simulink model "Singlephase_INC_grid"  (R2023b)
settings: Solver=ode23t  StartTime=0.0  StopTime=4  FixedStep=1e-5  MaxStep=1e-4  RelTol=10e-4  EnableMultiTasking=on
undefined symbols (not defined in the file): Ion, Lithium, sigbuilder_block
libraries: spsFirstOrderFilterLib x13, spsSeriesRLCBranchLib x12, spsCurrentMeasurementLib x9, spsIGBTDiodeLib x7, spsVoltageMeasurementLib x5, spsPWMGeneratorDCDCLib x3, powerlib_extras x3, spsThreePhaseVIMeasurementLib x2, spsDiodeLib x2, spsGroundLib x2, spspowerguiLib x2, spsBatteryLib x1
settings Model: Creator=Administrator  LastModifiedBy=Chani
settings SolverCC: ZeroCrossControl=DisableAll  AlgebraicLoopSolver=TrustRegion
settings DataIOCC: LimitDataPoints=on  SaveFormat=Array  SignalLoggingSaveFormat=ModelDataLogs  ReturnWorkspaceOutputs=off
settings OptimizationCC: ExpressionDepthLimit=2147483647  LifeSpan=inf
settings DebuggingCC: UnderspecifiedInitializationDetection=Classic  MergeDetectMultiDrivingBlocksExec=none  SolverPrmCheckMsg=warning  FcnCallInpInsideContextMsg=warning  UnconnectedInputMsg=warning  UnconnectedOutputMsg=warning  UnconnectedLineMsg=warning  StateNameClashWarn=warning  SFUnexpectedBacktrackingDiag=warning  SFNoUnconditionalDefaultTransitionDiag=warning  SFExecutionAtInitializationDiag=none  ArithmeticOperatorsInVariantConditions=warning
settings HardwareCC: ProdBitPerPointer=32  ProdBitPerSizeT=32  ProdBitPerPtrDiffT=32  ProdLargestAtomicFloat=None  ProdIntDivRoundTo=Undefined  ProdEndianess=Unspecified  ProdWordSize=32  ProdHWDeviceType=32-bit Generic
settings ModelReferenceCC: EnableRefExpFcnMdlSchedulingChecks=on  PropagateSignalLabelsOutOfModel=off
settings SFSimCC: SimUseLocalCustomCode=off  CustomCodeUndefinedFunction=UseInterfaceOnly
settings RTWCC: RTWUseLocalCustomCode=off
settings CodeAppCC: StateflowObjectComments=on
settings GRTTargetCC: TargetLangStandard=C89/C90 (ANSI)  CombineOutputUpdateFcns=off  GRTInterface=on
settings ConfigComp: CovMetricSettings=dw  CovSaveCumulativeToWorkspaceVar=on  CovSaveSingleToWorkspaceVar=on  CovExternalEMLEnable=off
settings SimscapeCC: SimscapeNormalizeSystem=off

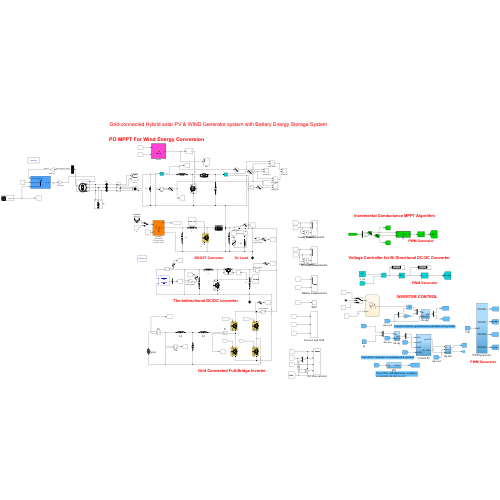
[thumbnail: Simulink's stored preview of the top-level diagram]
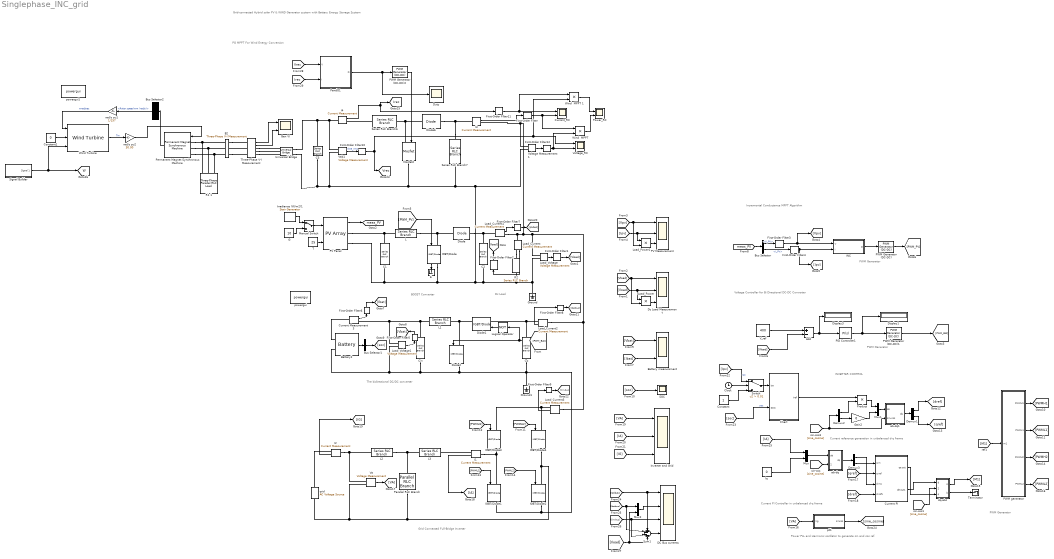
== system Singlephase_INC_grid ==
  note: Grid-connected Hybrid solar PV & WIND Generator system with Battery Energy Storage System
  note: Dc Load
  note: BOOST Converter
  note: Incremental Conductance MPPT Algorithm
  note: PWM Generator
  note: The bidirectional DC/DC converter
  note: PWM Generator
  note: Voltage Controller for Bi Directional DC-DC Converter
  note: Grid Connected Full-Bridge Inverter
  note: Current PI Controller in unbalanced d-q frame
  note: Power PLL and Harmonic oscillator to generate sin and cos ref.
  note: INVERTER CONTROL
  note: Current reference generation in unbalanced d-q frame
  note: PWM Generator
  note: PO MPPT For Wind Energy Conversion
  Add : Sum  Inputs=+-
  "B2 " : spsThreePhaseVIMeasurementLib/Three-Phase V-I Measurement  VoltageMeasurement=no  SetLabelV=on  LabelV=Vabc_B2  Vpu=off  VpuLL=off  CurrentMeasurement=no  SetLabelI=on  LabelI=Iabc_B2  Ipu=off  Pbase=100e6  Vbase=500e3  OutputType=Magnitude  PhasorSimulation=off  PSBequivalent=0
  Battery measurement : Scope  NumInputPorts=2
  Battery2 : spsBatteryLib/Battery  BatType=Lithium-Ion  ShowTempParam=off  ThermalPreset=no  ShowAgeParam=off  NomV=12*20  NomQ=48  SOC=50  Batt_Tr=0.0001  PresetModel=on  MaxQ=48  MinV=180  FullV=279.3569  Dis_rate=20.8696  R=0.05  Normal_OP=43.4087  expZone="[259.2926      2.358261]"  current=[1.5 3]  Units=Ampere-hour  Tci=20  NomT=20  T2=-30  MaxQ2=4.8  FullV2=7.1  Normal_OP2=5.72  expZone2="[6.58  1]"  Rca=0.6  ti=1000  Dp=0  Neq0=0  Tsim=1e6  Ta1=25  Qeol=5.4*0.9  Reol=0.013333*1.2  Char_age=[2.3478, 3]  Dis_age=[2.3478, 10]  N1=1500  N2=10500  N3=1000  N4=1400  Ta2=45  N5=950
      settings: LibrarySourceBlock=electricdrivelib/Extra Sources/Battery
  Bus Selector : BusSelector  OutputSignals=V_PV,I_PV
  Bus Selector1 : BusSelector  OutputSignals=SOC (%)  OutputAsBus=on
  Bus Selector2 : BusSelector  OutputSignals=Rotor speed wm (rad/s)
  C1 : spsSeriesRLCBranchLib/Series RLC Branch  LConnTagsString=__new0  RConnTagsString=__new0  BranchType=C  Resistance=1  Inductance=1e-3  SetiL0=off  InitialCurrent=0  Capacitance=4.8250e-05  Setx0=off  InitialVoltage=0  Measurements=None
  C2 : spsSeriesRLCBranchLib/Series RLC Branch  LConnTagsString=__new0  RConnTagsString=__new0  BranchType=C  Resistance=1  Inductance=1e-3  SetiL0=off  InitialCurrent=0  Capacitance=4.8250e-05  Setx0=off  InitialVoltage=0  Measurements=None
  C3 : spsSeriesRLCBranchLib/Series RLC Branch  LConnTagsString=__new0  RConnTagsString=__new0  BranchType=C  Resistance=0.001  Inductance=1e-3  SetiL0=off  InitialCurrent=0  Capacitance=4.8250e-05  Setx0=off  InitialVoltage=0  Measurements=None
  Chart : Stateflow chart  TreatAsAtomicUnit=on
  Cin : spsSeriesRLCBranchLib/Series RLC Branch  LConnTagsString=__new0  RConnTagsString=__new0  BranchType=C  Resistance=1  Inductance=3e-3  SetiL0=off  InitialCurrent=0  Capacitance=4.8250e-05  Setx0=off  InitialVoltage=0  Measurements=None
  Clock : Clock
  Co : spsSeriesRLCBranchLib/Series RLC Branch  LConnTagsString=__new0  RConnTagsString=__new0  BranchType=C  Resistance=1  Inductance=3e-3  SetiL0=off  InitialCurrent=0  Capacitance=4.8250e-05  Setx0=off  InitialVoltage=0  Measurements=None
  Constant : Constant
  Constant1 : Constant  Value=0
  Current Measurement3 : spsCurrentMeasurementLib/Current Measurement  PhasorSimulation=off  OutputType=Complex  PSBequivalent=0
  Current PI : Subsystem
  Current_RC : Scope  NumInputPorts=2
  DC Bus currents : Scope  NumInputPorts=4
  Dc Load Measurement : Scope  NumInputPorts=3
  Demux1 : Demux  Outputs=2
  Demux2 : Demux  Outputs=2
  Demux3 : Demux  Outputs=2
  Diode : spsDiodeLib/Diode  Ron=0.001  Lon=0  Vf=0.8  IC=0  UseSnubber=off  Rs=500  Cs=250e-9  Measurements=off
  Diode1 : spsIGBTDiodeLib/IGBT//Diode  Ron=1e-3  Rs=1e5  Cs=inf  Measurements=on
  Diode2 : spsIGBTDiodeLib/IGBT//Diode  Ron=1e-3  Rs=1e5  Cs=inf  Measurements=on
  Diode6 : spsDiodeLib/Diode  Ron=0.001  Lon=0  Vf=0.8  IC=0  UseSnubber=0  Rs=500  Cs=250e-9  Measurements=off
  Display1 : Display
  Display3 : Display
  Duty : Scope
  E : Terminator
  First-Order Filter{,1..12} (13 alike) : spsFirstOrderFilterLib/First-Order Filter  FilterType=Lowpass  Tc=10e-3  Ts=0  Initialize=on  Vac_Init=[0, 0, 60]  Vdc_Init=0  PlotResponse=off  FreqRange="[0,  200,  1]"
  G : Constant  Value=10
  Gain2 : Gain  Gain=0
  Gen VI : Scope  NumInputPorts=2
  Ground : spsGroundLib/Ground  LConnTagsString=a
  Ground1 : spsGroundLib/Ground  LConnTagsString=a
  I{1..4} (4 alike) : spsCurrentMeasurementLib/Current Measurement  PhasorSimulation=off  OutputType=Complex  PSBequivalent=0
  IGBT/Diode{,1..4} (5 alike) : spsIGBTDiodeLib/IGBT//Diode  Ron=1e-3  Rs=1e5  Cs=inf  Measurements=on
  INC : MATLAB Function  TreatAsAtomicUnit=on
  Inverter and Grid : Scope  NumInputPorts=3
  Iq : Constant  Value=0
  Irradiance (W/m2)1 : spsStairGeneratorLib/Stair Generator  t=[0, 0.3, 0.6,0.9, 1.2]  e=[1,0.5, 0.01, 0.5, 1]*1000  Ts=0.0001
  L : spsSeriesRLCBranchLib/Series RLC Branch  LConnTagsString=__new0  RConnTagsString=__new0  BranchType=L  Resistance=1  Inductance=0.1164  SetiL0=off  InitialCurrent=0  Capacitance=1e-6  Setx0=off  InitialVoltage=0  Measurements=None
  L1 : spsSeriesRLCBranchLib/Series RLC Branch  LConnTagsString=__new0  RConnTagsString=__new0  BranchType=L  Resistance=.25  Inductance=0.1164  SetiL0=off  InitialCurrent=0  Capacitance=1e-6  Setx0=off  InitialVoltage=0  Measurements=None
  L2 : spsSeriesRLCBranchLib/Series RLC Branch  LConnTagsString=__new0  RConnTagsString=__new0  BranchType=L  Resistance=0.001  Inductance=0.72e-3  SetiL0=off  InitialCurrent=0  Capacitance=1e-6  Setx0=off  InitialVoltage=0  Measurements=None
  L3 : spsSeriesRLCBranchLib/Series RLC Branch  LConnTagsString=__new0  RConnTagsString=__new0  BranchType=L  Resistance=1.5  Inductance=6.6e-3  SetiL0=off  InitialCurrent=0  Capacitance=1e-6  Setx0=off  InitialVoltage=0  Measurements=None
  Load_Current{,1..3} (4 alike) : spsCurrentMeasurementLib/Current Measurement  PhasorSimulation=off  OutputType=Complex  PSBequivalent=0
  Load_Power : Product  RndMeth=Zero
  Load_Power1 : Product  RndMeth=Zero
  Load_Voltage : spsVoltageMeasurementLib/Voltage Measurement  PhasorSimulation=off  OutputType=Complex  PSBequivalent=0
  Load_Voltage1 : spsVoltageMeasurementLib/Voltage Measurement  PhasorSimulation=off  OutputType=Complex  PSBequivalent=0
  Logical Operator : Logic  Operator=NOT  AllPortsSameDT=off  OutDataTypeStr=boolean
  Manual Switch : ManualSwitch
  Mosfet2 : spsMosfetLib/Mosfet  Ron=0.1  Lon=0  Rd=0.01  Vfd=0.8  IC=0  Rs=1e5  Cs=inf  Measurements=off
  Mux : Mux  Inputs=2
  Mux1 : Mux  Inputs=2
  Mux2 : Mux  Inputs=2
  PID Controller1 : slpidlib/PID Controller  Controller=PI  Form=Parallel  TimeDomain=Continuous-time  UseExternalTs=off  SampleTime=-1  IntegratorMethod=Forward Euler  FilterMethod=Forward Euler  ControllerParametersSource=internal  P=0.00001  I=0.05  UseKiTs=off  D=0  N=100  UseFilter=on  TunerSelectOption=Transfer Function Based (PID Tuner App)  InitialConditionSource=internal  InitialConditionForIntegrator=0  InitialConditionForFilter=0  DifferentiatorICPrevScaledInput=0  ExternalReset=none  TrackingMode=off  Kt=1  LimitOutput=off  SatLimitsSource=internal  UpperSaturationLimit=inf  LowerSaturationLimit=-inf  LinearizeAsGain=on  AntiWindupMode=none  Kb=1  LimitIntegrator=off  UpperIntegratorSaturationLimit=inf  LowerIntegratorSaturationLimit=-inf  POutMin=[]  POutMax=[]  IOutMin=[]  IOutMax=[]  DOutMin=[]  DOutMax=[]  NOutMin=[]  NOutMax=[]  SumOutMin=[]  SumOutMax=[]  SaturationOutMin=[]  SaturationOutMax=[]  PParamMin=[]  PParamMax=[]  IParamMin=[]  IParamMax=[]  DParamMin=[]  DParamMax=[]  NParamMin=[]  NParamMax=[]  KbParamMin=[]  KbParamMax=[]  KtParamMin=[]  KtParamMax=[]  KbOutMin=[]  KbOutMax=[]  KtOutMin=[]  KtOutMax=[]  IntegratorOutMin=[]  IntegratorOutMax=[]  FilterOutMin=[]  FilterOutMax=[]  SumI1OutMin=[]  SumI1OutMax=[]  SumI2OutMin=[]  SumI2OutMax=[]  SumI3OutMin=[]  SumI3OutMax=[]  SumI4OutMin=[]  SumI4OutMax=[]  SumDOutMin=[]  SumDOutMax=[]  DifferentiatorOutMin=[]  DifferentiatorOutMax=[]  FilterDiffOutCoefMin=[]  FilterDiffOutCoefMax=[]  ReciprocalOutMin=[]  ReciprocalOutMax=[]  SumDenOutMin=[]  SumDenOutMax=[]  SumNumOutMin=[]  SumNumOutMax=[]  DivideOutMin=[]  DivideOutMax=[]  UdiffTsProdOutMin=[]  UdiffTsProdOutMax=[]  NTsProdOutMin=[]  NTsProdOutMax=[]  UintegralTsProdOutMin=[]  UintegralTsProdOutMax=[]  UngainTsProdOutMin=[]  UngainTsProdOutMax=[]  ClampingZeroOutDataTypeStr=Inherit: Inherit via back propagation  ClampingZeroOutMin=[]  ClampingZeroOutMax=[]  FilterDenConstantOutDataTypeStr=Inherit: Inherit via back propagation  FilterDenConstantOutMin=[]  FilterDenConstantOutMax=[]  PCopyOutDataTypeStr=Inherit: Inherit via back propagation  PCopyOutMin=[]  PCopyOutMax=[]  NCopyOutDataTypeStr=Inherit: Inherit via back propagation  NCopyOutMin=[]  NCopyOutMax=[]  IntegratorContinuousStateAttributes=''  IntegratorStateMustResolveToSignalObject=off  IntegratorRTWStateStorageClass=Auto  FilterContinuousStateAttributes=''  FilterStateMustResolveToSignalObject=off  FilterRTWStateStorageClass=Auto  ParallelPVariant=InternalParameters  IdealPVariant=Disabled  IVariant=InternalParameters  DVariant=Disabled  IntegratorVariant=Continuous  SatVariant=Disabled  AWVariant=Passthrough  PCopyVariant=Disabled  TRVariant=Disabled  FdbkBlocksVariant=Forward  IdealPFdbkVariant=Disabled  SatFdbkVariant=Disabled  DerivativeFilterVariant=Disabled  NVariant=Disabled  NCopyVariant=Disabled_SignalSpec  FilterICVariant=Disabled  IntegratorICVariant=InternalICs  ExternalResetVariant=Disabled  TRSumVariant=Passthrough  SumFdbkVariant=Disabled  SumVariant=Sum_PI  TsampFilterVariant=InternalTs  TsampNgainVariant=Passthrough  TsampIntegralVariant=Disabled_SignalSpec  ExternalSaturationOutDataTypeStr=Inherit: Same as second input
  PV Measurement : Scope  NumInputPorts=3
  PV Panel : spsPVArrayLib/PV Array  Npar=1  Nser=8  PlotType=array @ 25 deg.C & specified irradiances  S_vec="[ 1000 800  600  400 ]"  Temp_C_vec="[ 45 25  ]"  ModuleName=User-defined  PlotWhenSelected=off  Pm=250.205  Ncell=60  Voc=37.3  Isc=8.66  Vm=30.7  Im=8.15  beta_Voc_pc=-0.36901  alpha_Isc_pc=0.086998  beta_Voc=-0.13764  alpha_Isc=0.007534  IL=8.7062  I0=4.1579e-10  nI=1.0189  Rsh=240.6015  Rs=0.23732  RobustModel=off  RobustCellTemperature=313.3991  BAL=on  Tc=1e-6  Tfilter=1e-5
      settings: AttributesFormatString=|
      | %<ModuleName>
      | %<Nser>-module string
      | %<Npar> parallel strings
  PWM Generator (DC-DC) : spsPWMGeneratorDCDCLib/PWM Generator (DC-DC)  Fsw=10000  Ts=0
  PWM Generator (DC-DC)1 : spsPWMGeneratorDCDCLib/PWM Generator (DC-DC)  Fsw=10000  Ts=0
  PWM Generator (DC-DC)2 : spsPWMGeneratorDCDCLib/PWM Generator (DC-DC)  Fsw=5000  Ts=0
  PWM generator : Subsystem
  PandO1 : MATLAB Function  TreatAsAtomicUnit=on
  Parallel RLC Branch : spsParallelRLCBranchLib/Parallel RLC Branch  LConnTagsString=a  RConnTagsString=__new0  BranchType=C  Resistance=1  Inductance=1e-3  SetiL0=off  InitialCurrent=0  Capacitance=6.91e-6  Setx0=off  InitialVoltage=0  Measurements=None
  Permanent Magnet Synchronous Machine : spsPermanentMagnetSynchronousMachineLib/Permanent Magnet Synchronous Machine  NbPhases=3  FluxDistribution=Sinusoidal  RotorType=Round  MechanicalLoad=Torque Tm  PresetModel="06:  10 Nm 300 Vdc 2300 RPM - 14.2 Nm"  ShowDetailedParameters=on  MeasurementBus=off  Resistance=0.4578  Inductance=8.5e-3  dqInductances=[8.5e-3,8.5e-3]  La=0.00334  MachineConstant=Flux linkage established by magnets (V.s)  Flux=0.171  VoltageCst=124.0639  TorqueCst=1.026  Flat=120  Mechanical=[0.001469 0.0003035 4 0]  PolePairs=4  InitialConditions=[0,0, 0,0]  InitialConditions5ph=[0 0 0 0 0 0]  RefAngle=90 degrees behind phase A axis (modified Park)  IterativeDiscreteModel=Trapezoidal non iterative  TsBlock=-1  TsPowergui=0
  Power_RC : Scope  NumInputPorts=2
  Product : Product  RndMeth=Zero
  R1 1 : spsThreePhaseParallelRLCLoadLib/Three-Phase Parallel RLC Load  LConnTagsString=A|B|C  Configuration=Y (grounded)  NominalVoltage=220  Vabc=[1e3 1e3 1e3]  Vabcp=[1e3 1e3 1e3]  NominalFrequency=50  UnbalancedPower=off  ActivePower=1000  InductivePower=0  CapacitivePower=0  Pabc=[9e3 9e3 9e3]  QLabc=[100 90 110]  QCabc=[100 90 110]  Pabcp=[10e3 9e3 11e3]  QLabcp=[100 90 110]  QCabcp=[100 90 110]  Measurements=None  LoadType=constant Z
  R2 : spsSeriesRLCBranchLib/Series RLC Branch  LConnTagsString=__new0  RConnTagsString=__new0  BranchType=R  Resistance=160  Inductance=1e-3  SetiL0=off  InitialCurrent=0  Capacitance=1e-6  Setx0=off  InitialVoltage=0  Measurements=None
  SOC : Scope
  Series RLC Branch6 : spsSeriesRLCBranchLib/Series RLC Branch  LConnTagsString=__new0  RConnTagsString=__new0  BranchType=L  Resistance=1  Inductance=0.1164  SetiL0=off  InitialCurrent=0  Capacitance=1e-6  Setx0=off  InitialVoltage=0  Measurements=None
  Series RLC Branch7 : spsSeriesRLCBranchLib/Series RLC Branch  LConnTagsString=__new0  RConnTagsString=__new0  BranchType=C  Resistance=110  Inductance=1e-3  SetiL0=off  InitialCurrent=0  Capacitance=4.8250e-05  Setx0=off  InitialVoltage=0  Measurements=None
  Signal Builder : Subsystem  Tag=STV Subsys  LoadFcn=sigbuilder_block('load');  StartFcn=sigbuilder_block('start');  StopFcn=sigbuilder_block('stop');  ClipboardFcn=sigbuilder_block('clipboard');  mask(Sigbuilder block){tuvar=[0:10]}
      mask help: Simulink:masks:SigbuilderBlock_MD
      mask init:
      | if ~strcmp(get_param(bdroot(gcbh),'SimulationStatus'),'stopped') tuvar = sigbuilder_block('maskInit'); end
      settings: CopyFcn=sigbuilder_block('copy');  DeleteFcn=sigbuilder_block('delete');  ModelCloseFcn=sigbuilder_block('modelClose');  PreSaveFcn=sigbuilder_block('preSave');  PauseFcn=sigbuilder_block('pause');  ContinueFcn=sigbuilder_block('continue');  NameChangeFcn=sigbuilder_block('namechange');  OpenFcn=sigbuilder_block('open',[333.75 182.25 550.5 359.25 ]);  CloseFcn=sigbuilder_block('close');
      mask Display: plot(0, 0, 100, 100,[2, 2, 32, 32, 2], [68, 8, 8, 68, 68],[32, 2], [38, 38], [32, 19, 2],[53, 60, 44], [32, 17, 17, 2],[16, 16, 31, 31]);txt = getActiveGroup(gcbh);text(2, 100, txt,'verticalAlignment', 'top');
  Sum1 : Sum  Inputs=+---
  Switch : Switch  Criteria=u2 > Threshold  Threshold=0.01  SaturateOnIntegerOverflow=off  InputSameDT=off
  T : Constant  Value=25
  Terminator : Terminator
  Three-Phase V-I Measurement : spsThreePhaseVIMeasurementLib/Three-Phase V-I Measurement  VoltageMeasurement=phase-to-phase  SetLabelV=off  LabelV=Vabc  Vpu=off  VpuLL=off  CurrentMeasurement=yes  SetLabelI=off  LabelI=Iabc  Ipu=off  Pbase=100e6  Vbase=500e3  OutputType=Complex  PhasorSimulation=off  PSBequivalent=0
  Universal Bridge : spsUniversalBridgeLib/Universal Bridge  Arms=3  SnubberResistance=1e5  SnubberCapacitance=inf  Device=Diodes  Ron=1e-3  Lon=0  ForwardVoltages="[  0  0  ]"  ForwardVoltage=0.8  GTOparameters=[ 10e-6 , 20e-6 ]  IGBTparameters=[ 1e-6 , 2e-6 ]  Measurements=None  Measurements_2=None  converterType=Rectifier
  V_ref : Constant  Value=400
  Va : spsVoltageMeasurementLib/Voltage Measurement  PhasorSimulation=off  OutputType=Complex  PSBequivalent=0
  Vab1 : spsVoltageMeasurementLib/Voltage Measurement  PhasorSimulation=off  OutputType=Complex  PSBequivalent=0
  Voltage Measurement1 : spsVoltageMeasurementLib/Voltage Measurement  PhasorSimulation=off  OutputType=Complex  PSBequivalent=0
  Voltage_RC : Scope  NumInputPorts=2
  "Wind  MPPT " : Product
  Wind  MPPT 1 : Product
  Wind Turbine : spsWindTurbineLib/Wind Turbine  Pnom=2.5e3  Pelec_base=2.5e3/0.9  wind_base=12  P_wind_base=1  speed_nom=1.3  pitch_angle=0  c1_c6="[0.51763          116          0.4            5           21     0.006795]"  cp_nom=0.48  lambda_nom=8.1
  ab-dq : Subsystem
  ab-dq1 : Subsystem
  dq-abc : Subsystem
  grid : spsACVoltageSourceLib/AC Voltage Source  Amplitude=230*sqrt(2)  Phase=0  Frequency=50  SampleTime=0  Measurements=None  BusType=swing  Pref=1e3  Qref=500  Qmin=-inf  Qmax=+inf
  pll1 : Subsystem
  powergui : spspowerguiLib/powergui  Priority=1  SimulationMode=Continuous  SampleTime=1e-6  frequency=60  Iterations=50  frequencyindice=0  Pbase=100e6  ErrMax=1e-4  UnitsV=kV  UnitsW=MW  buscounter=0  FunctionMessages=off  echomessages=off  EnableUseOfTLC=off  CurrentSourceSwitches=off  DisableSnubberDevices=off  DisableRonSwitches=off  DisableVfSwitches=off  DisplayEquations=off  AutomaticDiscreteSolvers=off  SolverType=Tustin/Backward Euler (TBE)  Interpol=off  ExternalGateDelay=off  methode=off  Ts=100  x0status=blocks  SPID=on  SwTol=0  HookPort=off  NonlinearTolerance=1e-4  nMaxIteration=100  ContinueOnMaxIteration=off  RestoreLinks=warning  ResistiveCurrentMeasurement=off  Frange=[0:2:500]  Ylog=off  Xlog=on  ShowGrid=off  save=off  variable=ZData  structure=0  ZoomFFT=off  StartTime=0.0  cycles=1  DisplayStyle=1  fundamental=60  FreqAxis=off  MaxFrequency=1000  frequencyindicesteady=1  RmsSteady=1  display=off
  powergui1 : spspowerguiLib/powergui  Priority=1  SimulationMode=Continuous  SampleTime=50e-6  frequency=60  Iterations=50  frequencyindice=0  Pbase=100e6  ErrMax=1e-4  UnitsV=kV  UnitsW=MW  buscounter=0  FunctionMessages=off  echomessages=off  EnableUseOfTLC=off  CurrentSourceSwitches=off  DisableSnubberDevices=off  DisableRonSwitches=off  DisableVfSwitches=off  DisplayEquations=off  AutomaticDiscreteSolvers=off  SolverType=Tustin/Backward Euler (TBE)  Interpol=off  ExternalGateDelay=off  methode=off  Ts=100  x0status=blocks  SPID=on  SwTol=0  HookPort=off  NonlinearTolerance=1e-4  nMaxIteration=100  ContinueOnMaxIteration=off  RestoreLinks=warning  ResistiveCurrentMeasurement=off  Frange=[0:2:500]  Ylog=off  Xlog=on  ShowGrid=off  save=off  variable=ZData  structure=0  ZoomFFT=off  StartTime=0.0  cycles=1  DisplayStyle=1  fundamental=60  FreqAxis=off  MaxFrequency=1000  frequencyindicesteady=1  RmsSteady=1  display=off
  rad/s pu1 : Gain  Gain=1/157  SaturateOnIntegerOverflow=on  OutDataTypeStr=Inherit: Same as input  ParamDataTypeStr=Inherit: Same as input
  rad/s pu2 : Gain  Gain=30.00  SaturateOnIntegerOverflow=on  OutDataTypeStr=Inherit: Same as input  ParamDataTypeStr=Inherit: Same as input
  tag scope: Irec=global, Vrec=global, W=global, meas_PV=global
  wires:
  T/1 -> PV Panel/2
  IGBT/Diode/1 -> E/1
  PV Panel/1 -> [meas_PV]
  [meas_PV] -> Bus Selector/1
  Bus Selector/2 -> First-Order Filter4/1  "<I_PV>"
  Bus Selector/1 -> First-Order Filter3/1  "<V_PV>"
  INC/1(D) -> PWM Generator (DC-DC)/1
  Manual Switch/1 -> PV Panel/1
  Irradiance (W/m2)1/1 -> Manual Switch/1
  G/1 -> Manual Switch/2
  V_ref/1 -> Add/1
  [Vload] -> Add/2
  Load_Voltage/1 -> First-Order Filter1/1
  Load_Current/1 -> First-Order Filter2/1
  First-Order Filter3/1 -> [Vpv], INC/1(V)
  First-Order Filter4/1 -> [Ipv], INC/2(I)
  Battery2/1 -> Bus Selector1/1
  Logical Operator/1 -> Diode1/1
  First-Order Filter2/1 -> [Iload]
  First-Order Filter1/1 -> [Vload]
  PWM Generator (DC-DC)/1 -> [PWM_PV]
  [PWM_PV] -> IGBT/Diode/1
  PWM Generator (DC-DC)1/1 -> [PWM_Bat]
  [PWM_Bat] -> Logical Operator/1, Diode2/1
  Current Measurement3/1 -> First-Order Filter6/1
  Load_Voltage1/1 -> First-Order Filter5/1
  Bus Selector1/1 -> [soc]
  [Vpv] -> Load_Power1/2, PV Measurement/1
  [Ipv] -> Load_Power1/1, PV Measurement/2
  Load_Power1/1 -> PV Measurement/3
  [Ibat] -> Battery measurement/2
  [Vbat] -> Battery measurement/1
  First-Order Filter6/1 -> [Ibat]
  First-Order Filter5/1 -> [Vbat]
  [Vload] -> Load_Power/2, Dc Load Measurement/1
  [Iload] -> Load_Power/1, Dc Load Measurement/2
  Load_Power/1 -> Dc Load Measurement/3
  [PWML1] -> IGBT/Diode1/1
  [PWML2] -> IGBT/Diode2/1
  [PWMH1] -> IGBT/Diode3/1
  [PWMH2] -> IGBT/Diode4/1
  Mux1/1 -> ab-dq1/1(ab)
  PWM generator/1(PWMH1) -> [PWMH1]
  ab-dq/1(dq) -> Demux3/1
  [VA] -> pll1/1(Vg)
  Current PI/1(qe out) -> dq-abc/3(q)
  Gain2/1 -> Mux1/2
  Product/1 -> Mux1/1
  Demux1/2 -> [qref]
  [dref] -> Current PI/4(d ref1)
  Demux2/2 -> Gain2/1
  Demux3/2 -> Current PI/1(q in)
  PWM generator/4(PWML2) -> [PWML2]
  [qref] -> Current PI/2(q ref)
  Demux2/1 -> Product/2
  [sine_cosine] -> ab-dq1/2(sin-cos), Demux2/1
  Iq/1 -> Mux/2
  Demux1/1 -> [dref]
  [sine_cosine] -> dq-abc/2(sin-cos)
  ab-dq1/1(dq) -> Demux1/1
  dq-abc/1(a) -> [M1]
  Mux/1 -> ab-dq/1(ab)
  [sine_cosine] -> ab-dq/2(sin-cos)
  PWM generator/3(PWMH2) -> [PWMH2]
  [IA] -> Mux/1
  Current PI/2(de out1) -> dq-abc/1(d)
  Demux3/1 -> Current PI/3(d in1)
  PWM generator/2(PWML1) -> [PWML1]
  pll1/1(sincos) -> [sine_cosine]
  [M1] -> PWM generator/1(m1)
  dq-abc/2(b) -> Terminator/1
  Va/1 -> [VA]
  I1/1 -> [IA]
  I2/1 -> [IG]
  [VA] -> Inverter and Grid/1
  [IA] -> Inverter and Grid/2
  [IG] -> Inverter and Grid/3
  [soc] -> SOC/1
  Add/1 -> PID Controller1/1, Display3/1
  PID Controller1/1 -> Display1/1, PWM Generator (DC-DC)1/1
  Load_Current1/1 -> First-Order Filter7/1
  Load_Current2/1 -> First-Order Filter8/1
  Load_Current3/1 -> First-Order Filter9/1
  [Ipvbus] -> Sum1/1, DC Bus currents/1
  [Iinvbus] -> Sum1/3, DC Bus currents/3
  First-Order Filter7/1 -> [Ipvbus]
  First-Order Filter8/1 -> [Ibatbus]
  First-Order Filter9/1 -> [Iinvbus]
  Sum1/1 -> DC Bus currents/4
  [Iload] -> Mux2/2, Sum1/4
  [Ibatbus] -> Sum1/2, Mux2/1
  Mux2/1 -> DC Bus currents/2
  [soc] -> Chart/2(SOC)  "soc"
  Chart/1(Iref) -> Product/1
  Switch/1 -> Chart/1(Ipv)
  Clock/1 -> Switch/2
  [Ipv] -> Switch/1  "Ipv"
  Constant/1 -> Switch/3
  I4/1 -> First-Order Filter11/1, [Irec]
  Constant1/1 -> Wind Turbine/2
  PWM Generator (DC-DC)2/1 -> Mosfet2/1
  Signal Builder/1(Signal 1) -> Wind Turbine/3, [W]
  [Irec] -> PandO1/2(I)
  First-Order Filter/1 -> "Wind  MPPT "/1, Current_RC/2
  Voltage Measurement1/1 -> First-Order Filter12/1
  First-Order Filter11/1 -> Wind  MPPT 1/1, Current_RC/1
  Vab1/1 -> First-Order Filter10/1  "Iline_rms"
  PandO1/1(D) -> Duty/1, PWM Generator (DC-DC)2/1
  "Wind  MPPT "/1 -> Power_RC/2
  Wind  MPPT 1/1 -> Power_RC/1
  rad/s pu1/1 -> Wind Turbine/1  "wrad/sec"
  rad/s pu2/1 -> Permanent Magnet Synchronous Machine/1
  Bus Selector2/1 -> rad/s pu1/1  "<Rotor speed wm (rad/s)>"
  [Vrec] -> PandO1/1(V)
  Three-Phase V-I Measurement/2 -> Gen VI/2
  I3/1 -> First-Order Filter/1
  Wind Turbine/1 -> rad/s pu2/1  "Tm"
  Three-Phase V-I Measurement/1 -> Gen VI/1
  Permanent Magnet Synchronous Machine/1 -> Bus Selector2/1
  First-Order Filter10/1 -> [Vrec], Wind  MPPT 1/2, Voltage_RC/1
  First-Order Filter12/1 -> "Wind  MPPT "/2, Voltage_RC/2
  connections:
  L/LConn1 -- PV Panel/RConn1 -- C1/RConn1
  L/RConn1 -- Diode/LConn1 -- IGBT/Diode/LConn1
  Diode/RConn1 -- Load_Current1/LConn1 -- C2/RConn1
  Current Measurement3/LConn1 -- Battery2/LConn1
  Load_Voltage1/LConn1 -- Current Measurement3/RConn1 -- L1/LConn1 -- Cin/LConn1
  Diode2/LConn1 -- Diode1/RConn1 -- L1/RConn1
  Load_Current/RConn1 -- R2/LConn1
  IGBT/Diode4/RConn1 -- IGBT/Diode2/LConn1 -- Parallel RLC Branch/RConn1 -- Va/LConn2 -- grid/LConn1
  IGBT/Diode3/RConn1 -- I1/LConn1 -- IGBT/Diode1/LConn1
  Load_Voltage1/LConn2 -- IGBT/Diode1/RConn1 -- IGBT/Diode2/RConn1 -- Ground1/LConn1 -- Co/RConn1 -- Diode2/RConn1 -- Cin/RConn1 -- Battery2/LConn2
  I1/RConn1 -- L3/RConn1
  Parallel RLC Branch/LConn1 -- L3/LConn1 -- L2/RConn1
  I2/LConn1 -- Va/LConn1 -- L2/LConn1
  I2/RConn1 -- grid/RConn1
  Co/LConn1 -- Load_Current2/RConn1 -- Diode1/LConn1
  IGBT/Diode3/LConn1 -- IGBT/Diode4/LConn1 -- Load_Current3/RConn1
  Load_Voltage/LConn2 -- Voltage Measurement1/LConn2 -- Series RLC Branch7/RConn1 -- Mosfet2/RConn1 -- Vab1/LConn2 -- C3/RConn1 -- Universal Bridge/RConn2 -- PV Panel/RConn2 -- C1/LConn1 -- IGBT/Diode/RConn1 -- C2/LConn1 -- R2/RConn1 -- Ground/LConn1
  Diode6/LConn1 -- Mosfet2/LConn1 -- Series RLC Branch6/RConn1
  R1 1/LConn1 -- Permanent Magnet Synchronous Machine/LConn1 -- "B2 "/LConn1
  R1 1/LConn3 -- Permanent Magnet Synchronous Machine/LConn3 -- "B2 "/LConn3
  R1 1/LConn2 -- Permanent Magnet Synchronous Machine/LConn2 -- "B2 "/LConn2
  I4/LConn1 -- Universal Bridge/RConn1 -- C3/LConn1 -- Vab1/LConn1
  Series RLC Branch7/LConn1 -- Diode6/RConn1 -- I3/LConn1
  Load_Current1/RConn1 -- Load_Current2/LConn1 -- Load_Current3/LConn1 -- Load_Voltage/LConn1 -- I3/RConn1 -- Voltage Measurement1/LConn1 -- Load_Current/LConn1
  Three-Phase V-I Measurement/LConn2 -- "B2 "/RConn2
  Three-Phase V-I Measurement/RConn1 -- Universal Bridge/LConn1
  Series RLC Branch6/LConn1 -- I4/RConn1
  "B2 "/RConn1 -- Three-Phase V-I Measurement/LConn1
  Three-Phase V-I Measurement/RConn3 -- Universal Bridge/LConn3
  Three-Phase V-I Measurement/RConn2 -- Universal Bridge/LConn2
  "B2 "/RConn3 -- Three-Phase V-I Measurement/LConn3

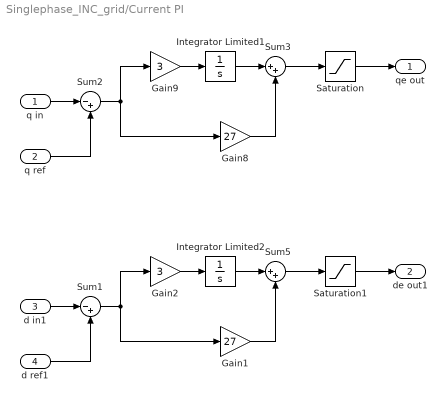
== system Singlephase_INC_grid/Current PI ==
  q in : Inport
  q ref : Inport  Port=2
  d in1 : Inport  Port=3
  d ref1 : Inport  Port=4
  Gain1 : Gain  Gain=27
  Gain2 : Gain  Gain=3
  Gain8 : Gain  Gain=27
  Gain9 : Gain  Gain=3
  Integrator Limited1 : Integrator  LimitOutput=on  UpperSaturationLimit=+5  LowerSaturationLimit=-5  ZeroCross=off
  Integrator Limited2 : Integrator  LimitOutput=on  UpperSaturationLimit=+5  LowerSaturationLimit=-5  ZeroCross=off
  Saturation : Saturate  UpperLimit=5  LowerLimit=-5
  Saturation1 : Saturate  UpperLimit=5  LowerLimit=-5
  Sum1 : Sum  Inputs=|-+
  Sum2 : Sum  Inputs=|-+
  Sum3 : Sum  Inputs=|++
  Sum5 : Sum  Inputs=|++
  qe out : Outport  VectorParamsAs1DForOutWhenUnconnected=off
  de out1 : Outport  Port=2  VectorParamsAs1DForOutWhenUnconnected=off
  wires:
  Gain8/1 -> Sum3/2
  Integrator Limited1/1 -> Sum3/1
  Sum2/1 -> Gain9/1, Gain8/1
  Gain9/1 -> Integrator Limited1/1
  q ref/1 -> Sum2/2
  q in/1 -> Sum2/1
  Gain1/1 -> Sum5/2
  Integrator Limited2/1 -> Sum5/1
  Sum1/1 -> Gain2/1, Gain1/1
  Gain2/1 -> Integrator Limited2/1
  d ref1/1 -> Sum1/2
  d in1/1 -> Sum1/1
  Sum3/1 -> Saturation/1
  Sum5/1 -> Saturation1/1
  Saturation/1 -> qe out/1
  Saturation1/1 -> de out1/1

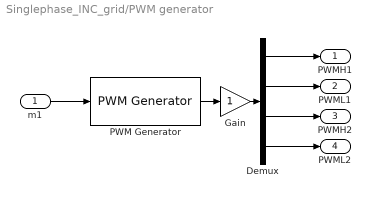
== system Singlephase_INC_grid/PWM generator ==
  m1 : Inport
  Demux : Demux
  Gain : Gain
  PWM Generator : powerlib_extras/Control  Blocks/PWM Generator  GeneratorMode="2-arm  bridge (4 pulses)"  Fc=7500  Internal=off  mIndex=0.4  Freq=60  Phase=0
  PWMH1 : Outport  VectorParamsAs1DForOutWhenUnconnected=off
  PWML1 : Outport  Port=2  VectorParamsAs1DForOutWhenUnconnected=off
  PWMH2 : Outport  Port=3  VectorParamsAs1DForOutWhenUnconnected=off
  PWML2 : Outport  Port=4  VectorParamsAs1DForOutWhenUnconnected=off
  wires:
  Gain/1 -> Demux/1
  PWM Generator/1 -> Gain/1
  Demux/2 -> PWML1/1
  Demux/1 -> PWMH1/1
  m1/1 -> PWM Generator/1
  Demux/3 -> PWMH2/1
  Demux/4 -> PWML2/1

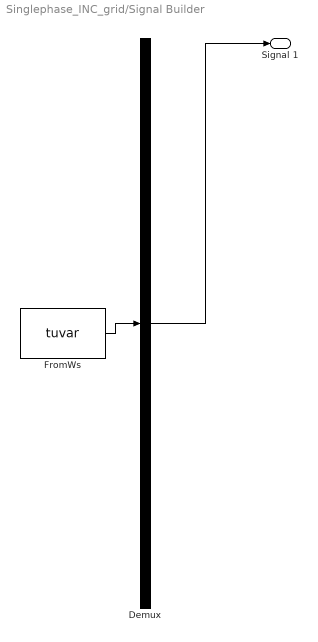
== system Singlephase_INC_grid/Signal Builder ==
  Demux : Demux  Tag=STV Demux  Outputs=1
      settings: DisplayOption=none
  FromWs : FromWorkspace  Tag=STV FromWs  VariableName=tuvar
      SigBuilderData=|
      | common.afterFinalStr = 'Extrapolate'
      | common.sampleTime = 0
      | dataSet.timeRange = [0 30]
      | dataSet.name = 'Group 1'
      | sbobj.Groups.Name = 'Group 1'
      | sbobj.Groups.Signals.Name = 'Signal 1'
      | sbobj.Groups.Signals.XData = [0 2 2 5 5 30]
      | sbobj.Groups.Signals.YData = [12 12 10.8 10.8 9.65 9.65]
      | sbobj.Groups.TimeRange = [0 30]
  Signal 1 : Outport  Tag=STV Outport  VectorParamsAs1DForOutWhenUnconnected=off
  wires:
  Demux/1 -> Signal 1/1
  FromWs/1 -> Demux/1

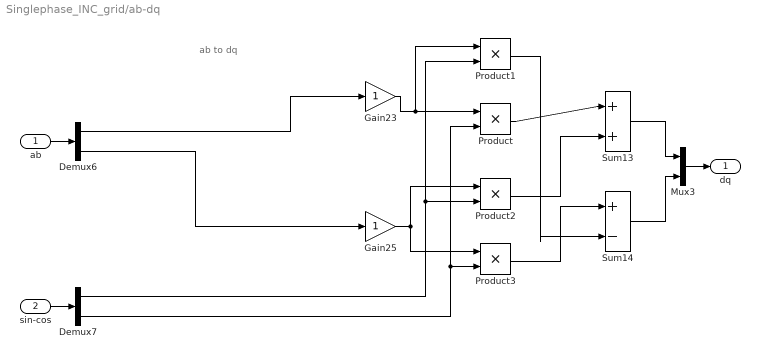
== system Singlephase_INC_grid/ab-dq ==
  note: ab to dq
  ab : Inport
  sin-cos : Inport  Port=2
  Demux6 : Demux  Outputs=2
  Demux7 : Demux  Outputs=2
  Gain23 : Gain
  Gain25 : Gain
  Mux3 : Mux  Inputs=2
  Product{,1..3} (4 alike) : Product  RndMeth=Zero
  Sum13 : Sum  Inputs=|++
  Sum14 : Sum  Inputs=|+-
  dq : Outport  VectorParamsAs1DForOutWhenUnconnected=off
  wires:
  Gain23/1 -> Product/1, Product1/1
  Demux7/2 -> Product/2, Product3/2
  Demux7/1 -> Product1/2, Product2/2
  Gain25/1 -> Product2/1, Product3/1
  Product/1 -> Sum13/1
  Product2/1 -> Sum13/2
  Product3/1 -> Sum14/1
  Product1/1 -> Sum14/2
  Sum13/1 -> Mux3/1
  Sum14/1 -> Mux3/2
  ab/1 -> Demux6/1
  Mux3/1 -> dq/1
  sin-cos/1 -> Demux7/1
  Demux6/2 -> Gain25/1
  Demux6/1 -> Gain23/1

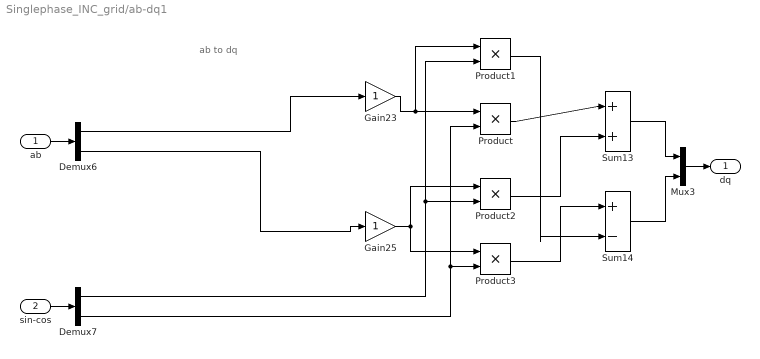
== system Singlephase_INC_grid/ab-dq1 ==
  note: ab to dq
  ab : Inport
  sin-cos : Inport  Port=2
  Demux6 : Demux  Outputs=2
  Demux7 : Demux  Outputs=2
  Gain23 : Gain
  Gain25 : Gain
  Mux3 : Mux  Inputs=2
  Product{,1..3} (4 alike) : Product  RndMeth=Zero
  Sum13 : Sum  Inputs=|++
  Sum14 : Sum  Inputs=|+-
  dq : Outport  VectorParamsAs1DForOutWhenUnconnected=off
  wires:
  Gain23/1 -> Product/1, Product1/1
  Demux7/2 -> Product/2, Product3/2
  Demux7/1 -> Product1/2, Product2/2
  Gain25/1 -> Product2/1, Product3/1
  Product/1 -> Sum13/1
  Product2/1 -> Sum13/2
  Product3/1 -> Sum14/1
  Product1/1 -> Sum14/2
  Sum13/1 -> Mux3/1
  Sum14/1 -> Mux3/2
  ab/1 -> Demux6/1
  Mux3/1 -> dq/1
  sin-cos/1 -> Demux7/1
  Demux6/2 -> Gain25/1
  Demux6/1 -> Gain23/1

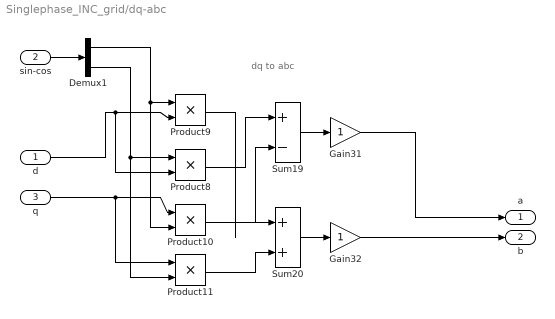
== system Singlephase_INC_grid/dq-abc ==
  note: dq to abc
  d : Inport
  sin-cos : Inport  Port=2
  q : Inport  Port=3
  Demux1 : Demux  Outputs=2
  Gain31 : Gain
  Gain32 : Gain
  Product{8..11} (4 alike) : Product  RndMeth=Zero
  Sum19 : Sum  Inputs=|+-
  Sum20 : Sum  Inputs=|++
  a : Outport  VectorParamsAs1DForOutWhenUnconnected=off
  b : Outport  Port=2  VectorParamsAs1DForOutWhenUnconnected=off
  wires:
  Sum19/1 -> Gain31/1
  Sum20/1 -> Gain32/1
  q/1 -> Product10/1, Product11/1
  d/1 -> Product9/2, Product8/2
  Product10/1 -> Sum19/2
  Product11/1 -> Sum20/2
  Product9/1 -> Sum20/1
  Product8/1 -> Sum19/1
  Demux1/1 -> Product10/2, Product9/1
  Demux1/2 -> Product11/2, Product8/1
  sin-cos/1 -> Demux1/1
  Gain31/1 -> a/1
  Gain32/1 -> b/1

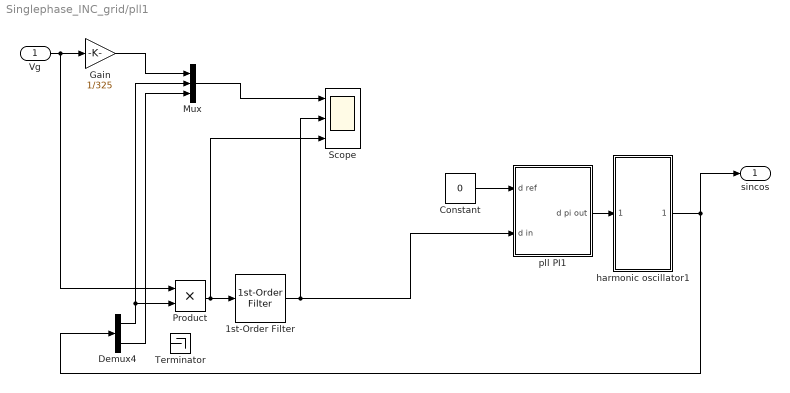
== system Singlephase_INC_grid/pll1 ==
  Vg : Inport
  1st-Order Filter : powerlib_extras/Control  Blocks/1st-Order  Filter  FilterType=Lowpass  Tc=50e-3  Initialize=off  Vac_Init=[0.8 -25 60]  Vdc_Init=-0.4  PlotResponse=off  param1=[1 500 1]
  Constant : Constant  Value=0
  Demux4 : Demux  Outputs=2
  Gain : Gain  Gain=1/325
  Mux : Mux  Inputs=3
  Product : Product  RndMeth=Zero
  Scope : Scope  NumInputPorts=3
  Terminator : Terminator
  harmonic oscillator1 : Subsystem
  pll PI1 : Subsystem
  sincos : Outport  VectorParamsAs1DForOutWhenUnconnected=off
  wires:
  pll PI1/1(d pi out) -> harmonic oscillator1/1(win 1)
  harmonic oscillator1/1(sin-cos) -> sincos/1, Demux4/1
  Demux4/1 -> Mux/2, Product/2
  Constant/1 -> pll PI1/1(d ref)
  Mux/1 -> Scope/1
  Gain/1 -> Mux/1
  Product/1 -> 1st-Order Filter/1, Scope/3
  1st-Order Filter/1 -> pll PI1/2(d in), Scope/2
  Demux4/2 -> Mux/3
  Vg/1 -> Gain/1, Product/1

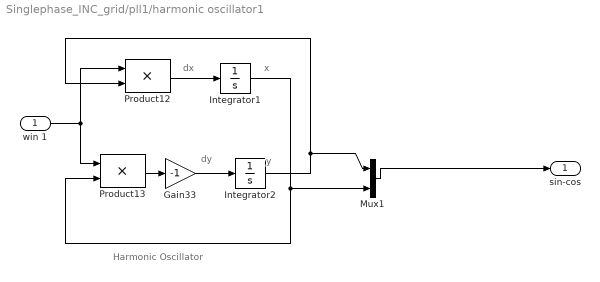
== system Singlephase_INC_grid/pll1/harmonic oscillator1 ==
  note: Harmonic Oscillator
  note: dy
  note: dx
  note: y
  note: x
  win 1 : Inport
  Gain33 : Gain  Gain=-1  SaturateOnIntegerOverflow=on  OutDataTypeStr=Inherit: Same as input  ParamDataTypeStr=Inherit: Same as input
  Integrator1 : Integrator  InitialCondition=1  LimitOutput=on  UpperSaturationLimit=1  LowerSaturationLimit=-1
  Integrator2 : Integrator  LimitOutput=on  UpperSaturationLimit=1  LowerSaturationLimit=-1
  Mux1 : Mux  Inputs=2
  Product12 : Product  SaturateOnIntegerOverflow=on  OutDataTypeStr=Inherit: Same as first input
  Product13 : Product  SaturateOnIntegerOverflow=on  OutDataTypeStr=Inherit: Same as first input
  sin-cos : Outport  VectorParamsAs1DForOutWhenUnconnected=off
  wires:
  win 1/1 -> Product13/1, Product12/1
  Gain33/1 -> Integrator2/1
  Product12/1 -> Integrator1/1
  Product13/1 -> Gain33/1
  Integrator1/1 -> Product13/2, Mux1/2
  Integrator2/1 -> Product12/2, Mux1/1
  Mux1/1 -> sin-cos/1

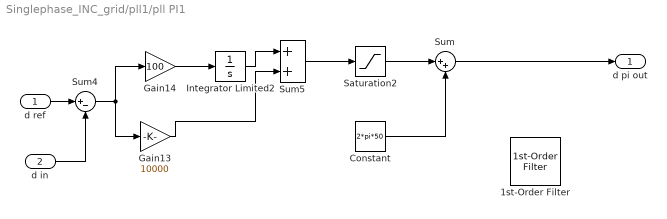
== system Singlephase_INC_grid/pll1/pll PI1 ==
  d ref : Inport
  d in : Inport  Port=2
  1st-Order Filter : powerlib_extras/Control  Blocks/1st-Order  Filter  FilterType=Lowpass  Tc=50e-3  Initialize=off  Vac_Init=[0.8 -25 60]  Vdc_Init=-0.4  PlotResponse=off  param1=[1 500 1]
  Constant : Constant  Value=2*pi*50
  Gain13 : Gain  Gain=10000
  Gain14 : Gain  Gain=100
  Integrator Limited2 : Integrator  LimitOutput=on  UpperSaturationLimit=4*pi*50  LowerSaturationLimit=-4*pi*50  ZeroCross=off
  Saturation2 : Saturate  UpperLimit=4*pi*50  LowerLimit=-4*pi*50  ZeroCross=off
  Sum : Sum  Inputs=|++
  Sum4 : Sum  Inputs=|+-
  Sum5 : Sum  Inputs=|++
  d pi out : Outport  VectorParamsAs1DForOutWhenUnconnected=off
  wires:
  Gain14/1 -> Integrator Limited2/1
  Sum4/1 -> Gain13/1, Gain14/1
  Sum5/1 -> Saturation2/1
  Integrator Limited2/1 -> Sum5/1
  Gain13/1 -> Sum5/2
  d ref/1 -> Sum4/1
  d in/1 -> Sum4/2
  Saturation2/1 -> Sum/1
  Constant/1 -> Sum/2
  Sum/1 -> d pi out/1

== matlab function Singlephase_INC_grid/PandO1 ==
  settings: updateMethod=DISCRETE
  data: D output; V input; I input

function D  = PandO(V, I)


Dinit = 0.5;  %Initial value for D output
Dmax = 0.6;   %Maximum value for D
Dmin = 0.45;   %Minimum value for D
deltaD = 0.0005; %Increment value used to increase/decrease the duty cycle D


persistent Vold Pold Dold;

dataType = 'double';

if isempty(Vold)
    Vold=0;
    Pold=0;
    Dold=Dinit;
end
P= V*I;
dV= V - Vold;
dP= P - Pold;

    if dP < 0
        if dV < 0
            D = Dold - deltaD;
        else
            D = Dold + deltaD;
        end
    else
        if dV < 0
            D = Dold + deltaD;
        else
            D = Dold - deltaD;
        end    
    end

if D >= Dmax | D<= Dmin
    D=Dold;
end

Dold=D;
Vold=V;
Pold=P;

== matlab function Singlephase_INC_grid/INC ==
  settings: updateMethod=DISCRETE
  data: D output; V input; I input
% author : Saad MOTAHHIR
% f= 10000hz (G)
function D  = INC(V, I)

Dinit = 0.42;  %Initial value for D output
Dmax = 0.95;   %Maximum value for D
Dmin = 0.01;   %Minimum value for D
deltaD = 0.000005; %Increment value used to increase/decrease the duty cycle D

  
persistent Vold Pold Dold M Iold;

dataType = 'double';

if isempty(Vold)
    Vold=0;
    Pold=0;
    Iold=0;
    Dold=Dinit;
    M=1;
end
P= V*I;
dV= V - Vold;
dP= P - Pold;
dI= I - Iold;
M=1;

if M < 0.005
    D=Dold;
else
    if dV == 0
        if dI == 0
            D=Dold;
        elseif dI>0
            D=Dold - (M*deltaD);
        else 
            D=Dold + (M*deltaD);
        end    
    else
        if dI/dV == -I/V
            D=Dold;
        elseif dI/dV>-I/V    
           D=Dold - (M*deltaD);
        else
           D=Dold + (M*deltaD);  
        end  
    end    
end

if D >= Dmax | D<= Dmin
    D=Dold;
end

Dold=D;
Vold=V;
Pold=P;
Iold=I;

== stateflow chart Singlephase_INC_grid/Chart ==
  state ToGrid
    entry:
    Iref=2
  state FromGrid
    entry:
    Iref=-10
  (default) -> ToGrid
  ToGrid -> FromGrid : [Ipv<0.5 && SOC<10]
  FromGrid -> ToGrid : [Ipv>0.5 && SOC>10]
  data: Ipv input; SOC input; Iref output
